simulink model "ForwardKinematics"  (R2022a)
settings: Solver=FixedStepDiscrete  StartTime=0.0  StopTime=inf  FixedStep=0.02  RelTol=1e-3
undefined symbols (not defined in the file or in its folder): w, x, y, z
libraries: ros2lib x2
settings Model: Creator=alessandrini  LastModifiedBy=alessandrini
settings OptimizationCC: EnhancedBackFolding=on  PassReuseOutputArgsAs=Individual arguments  ZeroExternalMemoryAtStartup=off  ZeroInternalMemoryAtStartup=off  MaxStackSize=64  OptimizeBlockOrder=speed  DifferentSizesBufferReuse=on  OptimizationCustomize=off  EfficientTunableParamExpr=on
settings DebuggingCC: ParameterTunabilityLossMsg=error
settings HardwareCC: ProdBitPerLong=64  ProdHWDeviceType=Intel->x86-64 (Linux 64)  UseEmbeddedCoderFeatures=off
settings SFSimCC: MATLABDynamicMemAlloc=off
settings RTWCC: SystemTargetFile=ert.tlc  HardwareBoard=Robot Operating System 2 (ROS 2)  TLCOptions="-aInlineSetEventsForThisBaseRateFcn=TLC_FALSE -aSuppressMultiTaskScheduler=TLC_FALSE  -aRateBasedStepFcn=0"  TemplateMakefile=ert_default_tmf  Toolchain=Colcon Tools  TargetLang=C++
settings CodeAppCC: ForceParamTrailComments=on  IgnoreCustomStorageClasses=off  OperatorAnnotations=on  SimulinkDataObjDesc=on  SFDataObjDesc=on  InsertBlockDesc=on
settings ERTTargetCC: CodeInterfacePackaging=C++ class  SupportNonInlinedSFcns=on  RootIOFormat=Structure reference

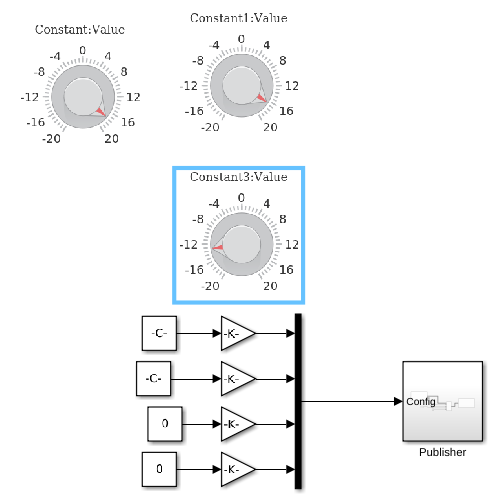
[thumbnail: Simulink's stored preview of the top-level diagram]
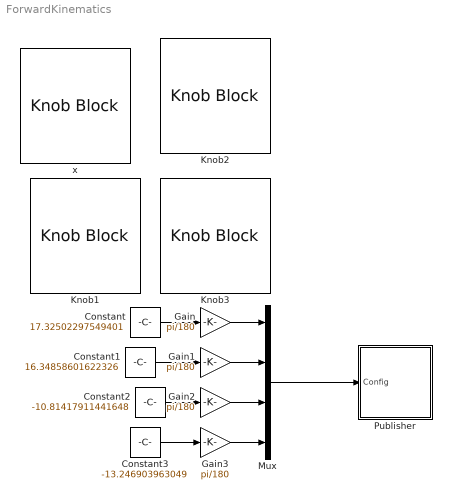
== system ForwardKinematics ==
  Constant : Constant  Value=17.32502297549401
  Constant1 : Constant  Value=16.34858601622326
  Constant2 : Constant  Value=-10.81417911441648
  Constant3 : Constant  Value=-13.246903963049
  Gain{,1..3} (4 alike) : Gain  Gain=pi/180
  Knob1 : KnobBlock  ScaleMin=-20  ScaleMax=20
  Knob2 : KnobBlock  ScaleMin=-20  ScaleMax=20
  Knob3 : KnobBlock  ScaleMin=-20  ScaleMax=20
  Mux : Mux
  Publisher : Subsystem
  x : KnobBlock  ScaleMin=-20  ScaleMax=20
  wires:
  Mux/1 -> Publisher/1(Config)
  Constant/1 -> Gain/1
  Constant3/1 -> Gain3/1
  Gain/1 -> Mux/1
  Gain1/1 -> Mux/2
  Gain2/1 -> Mux/3
  Gain3/1 -> Mux/4
  Constant1/1 -> Gain1/1
  Constant2/1 -> Gain2/1

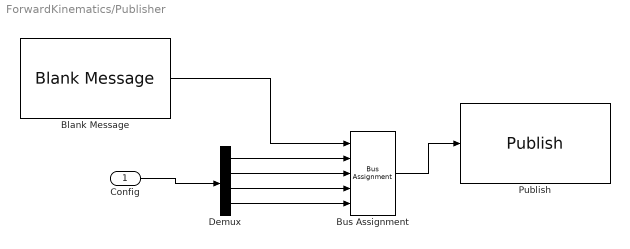
== system ForwardKinematics/Publisher ==
  Config : Inport
  Blank Message : ros2lib/Blank Message  messageClass=Message  entityType=geometry_msgs/Quaternion  messageType=geometry_msgs/Quaternion  SampleTime=0.02
      settings: SourceProductBaseCode=RR
  Bus Assignment : BusAssignment  AssignedSignals=x,y,z,w
  Demux : Demux
  Publish : ros2lib/Publish  topicSource=Specify your own  topic=Angles/ref  messageType=geometry_msgs/Quaternion  QOSHistory=Keep last  QOSDepth=1  QOSReliability=Reliable  QOSDurability=Volatile
      settings: SourceProductBaseCode=RR
  wires:
  Blank Message/1 -> Bus Assignment/1
  Bus Assignment/1 -> Publish/1
  Config/1 -> Demux/1
  Demux/1 -> Bus Assignment/2
  Demux/2 -> Bus Assignment/3
  Demux/3 -> Bus Assignment/4
  Demux/4 -> Bus Assignment/5
